simulink model "InterpolationQ_PDexample"  (R2019b)
settings: Solver=FixedStepDiscrete  StartTime=0.0  StopTime=13  FixedStep=0.01  MaxStep=0.01  RelTol=1e-3
undefined symbols (not defined in the file): DiscIntNeverNeededParam, Kd, Kp
libraries: simulink_extras x2, xpcutilitieslib x2, xpcrtudplib x2, simulink x1
settings Model: EnablePacing=on  Creator=Aljaz  LastModifiedBy=Aljaz
settings DataIOCC: SaveOutput=off  SaveTime=off  ReturnWorkspaceOutputs=off

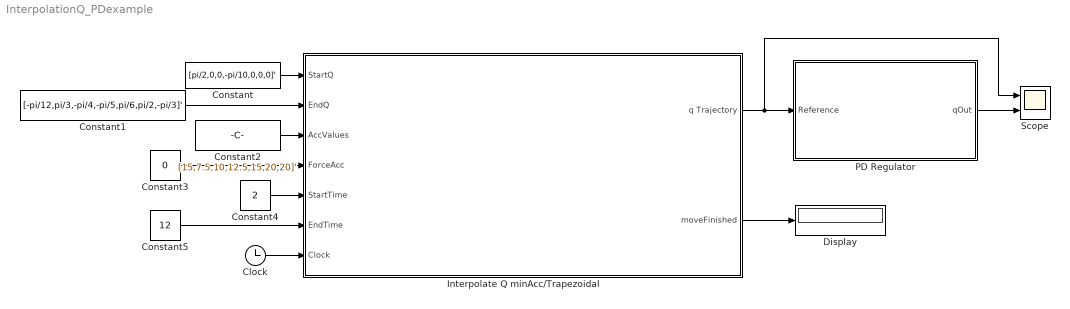
== system InterpolationQ_PDexample ==
  Clock : Clock
  Constant : Constant  Value=[pi/2,0,0,-pi/10,0,0,0]'
  Constant1 : Constant  Value=[-pi/12,pi/3,-pi/4,-pi/5,pi/6,pi/2,-pi/3]'
  Constant2 : Constant  Value=[15,7.5,10,12.5,15,20,20]'
  Constant3 : Constant  Value=0
  Constant4 : Constant  Value=2
  Constant5 : Constant  Value=12
  Display : Display
  Interpolate Q minAcc/Trapezoidal : Subsystem
  PD Regulator : Subsystem
  Scope : Scope  NumInputPorts=2
  wires:
  Interpolate Q minAcc/Trapezoidal/1(q Trajectory) -> Scope/1, PD Regulator/1(Reference)
  Interpolate Q minAcc/Trapezoidal/2(moveFinished) -> Display/1
  PD Regulator/1(qOut) -> Scope/2
  Constant/1 -> Interpolate Q minAcc/Trapezoidal/1(StartQ)
  Constant1/1 -> Interpolate Q minAcc/Trapezoidal/2(EndQ)
  Constant2/1 -> Interpolate Q minAcc/Trapezoidal/3(AccValues)
  Constant3/1 -> Interpolate Q minAcc/Trapezoidal/4(ForceAcc)
  Constant4/1 -> Interpolate Q minAcc/Trapezoidal/5(StartTime)
  Constant5/1 -> Interpolate Q minAcc/Trapezoidal/6(EndTime)
  Clock/1 -> Interpolate Q minAcc/Trapezoidal/7(Clock)

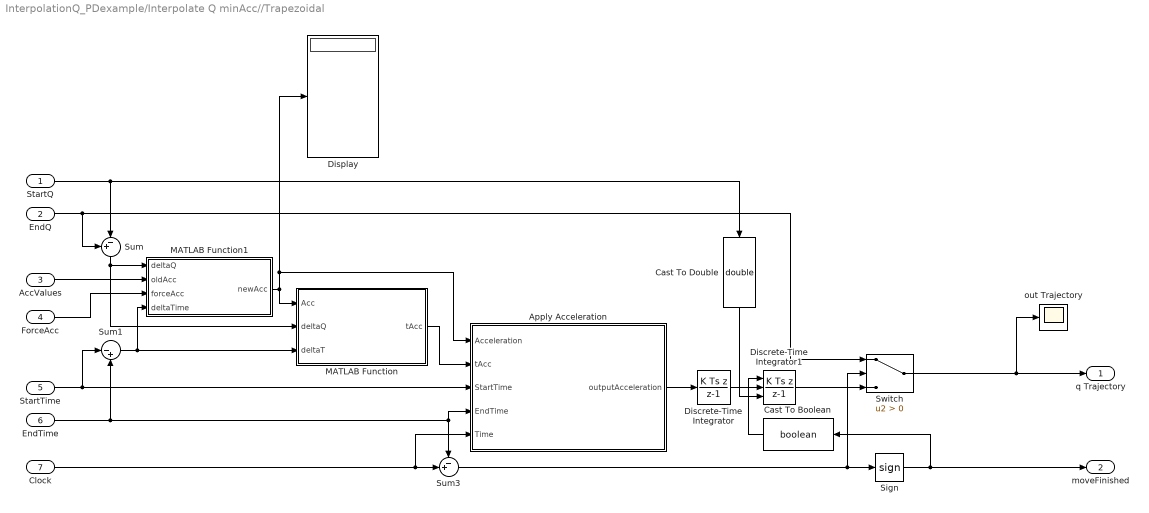
== system InterpolationQ_PDexample/Interpolate Q minAcc//Trapezoidal ==
  StartQ : Inport
  EndQ : Inport  Port=2
  AccValues : Inport  Port=3
  ForceAcc : Inport  Port=4
  StartTime : Inport  Port=5
  EndTime : Inport  Port=6
  Clock : Inport  Port=7
  Apply Acceleration : Subsystem
  Cast To Boolean : DataTypeConversion  OutDataTypeStr=boolean
  Cast To Double : DataTypeConversion  OutDataTypeStr=double
  Discrete-Time Integrator : DiscreteIntegrator  IntegratorMethod=Integration: Backward Euler  SampleTime=-1  ICPrevOutput=DiscIntNeverNeededParam  ICPrevScaledInput=DiscIntNeverNeededParam
  Discrete-Time Integrator1 : DiscreteIntegrator  IntegratorMethod=Integration: Backward Euler  ExternalReset=rising  InitialConditionSource=external  SampleTime=-1  ICPrevOutput=DiscIntNeverNeededParam  ICPrevScaledInput=DiscIntNeverNeededParam
  Display : Display
  MATLAB Function : MATLAB Function  TreatAsAtomicUnit=on
  MATLAB Function1 : MATLAB Function  TreatAsAtomicUnit=on
  Sign : Signum
  Sum : Sum  Inputs=+-|
  Sum1 : Sum  Inputs=|-+
  Sum3 : Sum  Inputs=-+|
  Switch : Switch  Criteria=u2 > Threshold
  out Trajectory : Scope
  q Trajectory : Outport
  moveFinished : Outport  Port=2
  wires:
  EndTime/1 -> Sum3/1, Apply Acceleration/4(EndTime), Sum1/2
  Sum3/1 -> Switch/2, Sign/1
  ForceAcc/1 -> MATLAB Function1/3(forceAcc)
  MATLAB Function/1(tAcc) -> Apply Acceleration/2(tAcc)
  Clock/1 -> Sum3/2, Apply Acceleration/5(Time)
  Sum1/1 -> MATLAB Function1/4(deltaTime), MATLAB Function/3(deltaT)
  AccValues/1 -> MATLAB Function1/2(oldAcc)
  StartQ/1 -> Cast To Double/1, Sum/2
  StartTime/1 -> Apply Acceleration/3(StartTime), Sum1/1
  Apply Acceleration/1(outputAcceleration) -> Discrete-Time Integrator/1
  Sum/1 -> MATLAB Function1/1(deltaQ), MATLAB Function/2(deltaQ)
  Discrete-Time Integrator/1 -> Discrete-Time Integrator1/1
  Discrete-Time Integrator1/1 -> Switch/3
  EndQ/1 -> Sum/1, Switch/1
  MATLAB Function1/1(newAcc) -> MATLAB Function/1(Acc), Display/1, Apply Acceleration/1(Acceleration)
  Sign/1 -> Cast To Boolean/1, moveFinished/1
  Switch/1 -> out Trajectory/1, q Trajectory/1
  Cast To Double/1 -> Discrete-Time Integrator1/3
  Cast To Boolean/1 -> Discrete-Time Integrator1/2

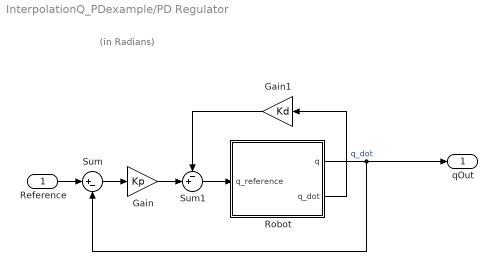
== system InterpolationQ_PDexample/PD Regulator ==
  note: (in Radians)
  Reference : Inport
  Gain : Gain  Gain=Kp
  Gain1 : Gain  Gain=Kd
  Robot : Subsystem
  Sum : Sum  Inputs=|+-
  Sum1 : Sum  Inputs=-+|
  qOut : Outport
  wires:
  Reference/1 -> Sum/1
  Sum1/1 -> Robot/1(q_reference)
  Gain/1 -> Sum1/2
  Sum/1 -> Gain/1
  Robot/1(q) -> qOut/1, Sum/2
  Gain1/1 -> Sum1/1
  Robot/2(q_dot) -> Gain1/1  "q_dot"

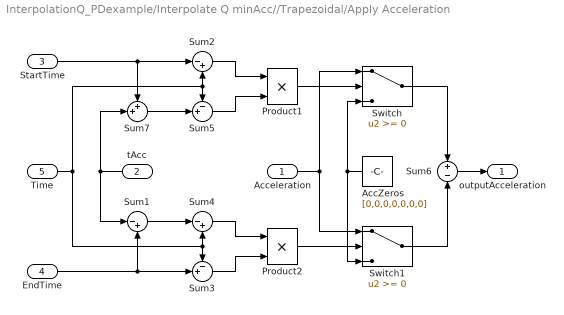
== system InterpolationQ_PDexample/Interpolate Q minAcc//Trapezoidal/Apply Acceleration ==
  Acceleration : Inport
  tAcc : Inport  Port=2
  StartTime : Inport  Port=3
  EndTime : Inport  Port=4
  Time : Inport  Port=5
  AccZeros : Constant  Value=[0,0,0,0,0,0,0]
  Product1 : Product
  Product2 : Product
  Sum1 : Sum  Inputs=|-+
  Sum2 : Sum  Inputs=|-+
  Sum3 : Sum  Inputs=-+|
  Sum4 : Sum  Inputs=|-+
  Sum5 : Sum  Inputs=-+|
  Sum6 : Sum  Inputs=+|-
  Sum7 : Sum  Inputs=++|
  Switch : Switch
  Switch1 : Switch
  outputAcceleration : Outport
  wires:
  Switch/1 -> Sum6/1
  Acceleration/1 -> Switch/1, Switch1/1
  Switch1/1 -> Sum6/2
  Product1/1 -> Switch/2
  AccZeros/1 -> Switch/3, Switch1/3
  Sum6/1 -> outputAcceleration/1
  Sum2/1 -> Product1/1
  Sum5/1 -> Product1/2
  Time/1 -> Sum4/2, Sum3/1, Sum2/2, Sum5/1
  StartTime/1 -> Sum7/1, Sum2/1
  tAcc/1 -> Sum1/1, Sum7/2
  Sum7/1 -> Sum5/2
  EndTime/1 -> Sum1/2, Sum3/2
  Sum1/1 -> Sum4/1
  Sum4/1 -> Product2/1
  Sum3/1 -> Product2/2
  Product2/1 -> Switch1/2

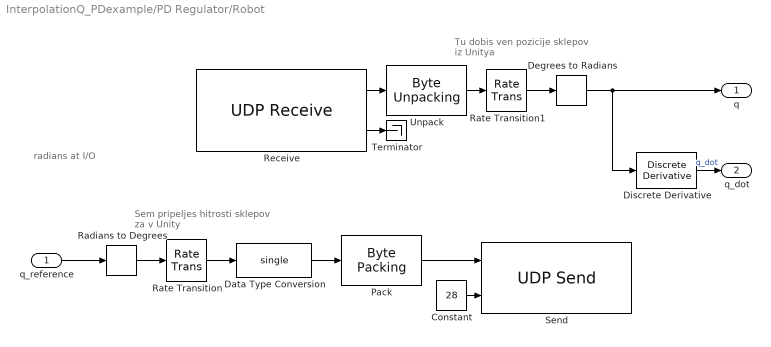
== system InterpolationQ_PDexample/PD Regulator/Robot ==
  note: radians at I/O
  note: Sem pripeljes hitrosti sklepov za v Unity
  note: Tu dobis ven pozicije sklepov iz Unitya
  q_reference : Inport
  Constant : Constant  Value=28
  Data Type Conversion : DataTypeConversion  OutDataTypeStr=single
  Degrees to Radians : simulink_extras/Transformations/Degrees to Radians
  Discrete Derivative : simulink/Discrete/Discrete Derivative  gainval=1  ICPrevScaledInput=0.0  OutMin=[]  OutMax=[]  OutDataType=fixdt(1, 16)  OutScaling=2^-10  DoSatur=off
  Pack : xpcutilitieslib/Byte Packing   MaskPackedDataType=uint8  MaskUnpackedDataTypes={'single'}  MaskAlignment=1
  Radians to Degrees : simulink_extras/Transformations/Radians to Degrees
  Rate Transition : RateTransition  InitialCondition=[0 0 0 0 0 0 0]
  Rate Transition1 : RateTransition
  Receive : xpcrtudplib/UDP Receive  ipAddressVal=Use host-target connection  localPort=25106  rcvWidth=7*4  rcvFmAny=off  fmAddress=127.0.0.1  rcvMulticast=off  multicastAddress={}  maxUDPQueue=8  sampleTime=0.01
      settings: SourceProductName=Simulink Real-Time
  Send : xpcrtudplib/UDP Send  ipAddressVal=Use host-target connection  localPort=-1  toAddress=127.0.0.1  toPort=25008  sampleTime=0.01
      settings: SourceProductName=Simulink Real-Time  SourceProductBaseCode=XP
  Terminator : Terminator
  Unpack : xpcutilitieslib/Byte Unpacking   MaskUnpackedDataTypes={'single'}  MaskUnpackedDataSizes={[7]}  MaskAlignment=1
      settings: SourceProductName=Simulink Real-Time  SourceProductBaseCode=XP
  q : Outport
  q_dot : Outport  Port=2
  wires:
  Constant/1 -> Send/2
  Pack/1 -> Send/1
  Receive/1 -> Unpack/1
  Rate Transition/1 -> Data Type Conversion/1
  Unpack/1 -> Rate Transition1/1
  Receive/2 -> Terminator/1
  Data Type Conversion/1 -> Pack/1
  Discrete Derivative/1 -> q_dot/1  "q_dot"
  Degrees to Radians/1 -> q/1, Discrete Derivative/1
  Rate Transition1/1 -> Degrees to Radians/1
  q_reference/1 -> Radians to Degrees/1
  Radians to Degrees/1 -> Rate Transition/1

== matlab function InterpolationQ_PDexample/Interpolate Q minAcc//Trapezoidal/MATLAB Function1 ==
  data: deltaQ input; oldAcc input; newAcc output; forceAcc input; deltaTime input
function newAcc = adjustAcc(deltaQ,oldAcc,forceAcc,deltaTime)
if forceAcc~=0
    newAcc=oldAcc.*sign(deltaQ); %adjust sign of acc
else
    tAcc=0.49*deltaTime;
    newAcc=(deltaQ./(deltaTime.*tAcc-tAcc.*tAcc));
end
end

== matlab function InterpolationQ_PDexample/Interpolate Q minAcc//Trapezoidal/MATLAB Function ==
  data: Acc input; deltaQ input; tAcc output; deltaT input
function tAcc = getAccTime(Acc,deltaQ,deltaT)

D=deltaT.^2.*Acc-4*deltaQ;
D=D./Acc;
tAcc=deltaT/2-0.5*sqrt(D);
end
